simulink model "Torque_Vectoring_Controller_dSpace"  (R2016a)
settings: Solver=FixedStepAuto  StartTime=0.0  StopTime=inf  FixedStep=car.dt  RelTol=1e-3
PostLoadFcn:
  | , if any(exist('dsrtsu_mdlpostloadfcn', 'file') == [2, 3, 6]), try dsrtsu_mdlpostloadfcn('Execute', bdroot); catch fprintf('Error in PostLoadFcn (dsrtsu_mdlpostloadfcn) for model "%s":\n %s\n', bdroot, lasterr); end, end,
InitFcn:
  | clear_close
  | dataCar
  | optParam
  | structSensors
  | structSettings
  | structEstimPar
  | structAero
  | structVariables
  | readFuzzyFile
StartFcn:
  | clear_close
  | dataCar
  | optParam
  | structSensors
  | structSettings
  | structEstimPar
  | structAero
  | structVariables
  | readFuzzyFile
undefined symbols (not defined in the file or in its folder): car, optPar
libraries: dsmpblib x23, fuzblock x1
(part 2 of 2)

== matlab function Torque_Vectoring_Controller_dSpace/Controls/Vehicle Estimated Parameters/Yaw Rate Reference ==
  data: sensors input; rref output; settings input; v input; car parameter
function rref = yawRateRef(sensors, settings, v, car)
if isempty(v); v =0;end
%Ackermann
wheelAngle = (sensors.wheelAngles(1)+sensors.wheelAngles(2))/2;
rref = wheelAngle*v/car.wb;




% 
% des_yaw_rate = vx*steering_angle / ...
%     (L_f + L_r + ...
%     m_chassis*vx^2*(L_r*(C_x_alpha_RL+C_x_alpha_RR)-L_f*(C_x_alpha_FL+C_x_alpha_FR))/...
%     ((C_x_alpha_RL+C_x_alpha_RR)*(C_x_alpha_FL+C_x_alpha_FR)*L));

== matlab function Torque_Vectoring_Controller_dSpace/Vehicle Sensors/Sensors ==
  data: ax input; sensors output Bus: sensorBus size=1; ay input; wheelspeed_FL input; wheelspeed_FR input; wheelspeed_RL input; wheelspeed_RR input; yawRate input; steeringAngle input; steerAngleFL input; steerAngleFR input; throttle input; brake input; torqueFL input; torqueFR input; torqueRL input; torqueRR input; ax_error input; ay_error input; yawRate_error input; knob1 input; knob2 input
function sensors = sensors(ax,ay,wheelspeed_FL,wheelspeed_FR,wheelspeed_RL,wheelspeed_RR,yawRate,steeringAngle,steerAngleFL,steerAngleFR, throttle,brake,torqueFL,torqueFR,torqueRL,torqueRR,ax_error,ay_error,yawRate_error,knob1,knob2)

sensors.ax = ax;
sensors.ay = ay;
sensors.wheelspeed = [wheelspeed_FL;wheelspeed_FR;wheelspeed_RL;wheelspeed_RR];
sensors.yawRate = yawRate;
sensors.steerAngle = steeringAngle;
sensors.wheelAngles = [steerAngleFL;steerAngleFR;0;0];
sensors.throttle = throttle;
sensors.brake= brake;
sensors.torque = [torqueFL;torqueFR;torqueRL;torqueRR];
sensors.ax_error = ax_error;
sensors.ay_error = ay_error;
sensors.yawRate_error = yawRate_error;
sensors.knob1 = knob1;
sensors.knob2 = knob2;
